simulink model "pmsm1"  (Simulink 7.0)
settings: Solver=ode23tb  StartTime=0.0  StopTime=1  MaxStep=1e-3  RelTol=1e-3
libraries: powerlib x12
settings Model: Creator=vegetable  LastModifiedBy=vegetable
settings OptimizationCC: InitFltsAndDblsToZero=off
settings DebuggingCC: SaveWithParameterizedLinksMsg=none  FcnCallInpInsideContextMsg=Enable All  StrictBusMsg=ErrorLevel1
settings HardwareCC: TargetHWDeviceType=32-bit Generic
settings GRTTargetCC: TargetFcnLib=ansi_tfl_tmw.mat

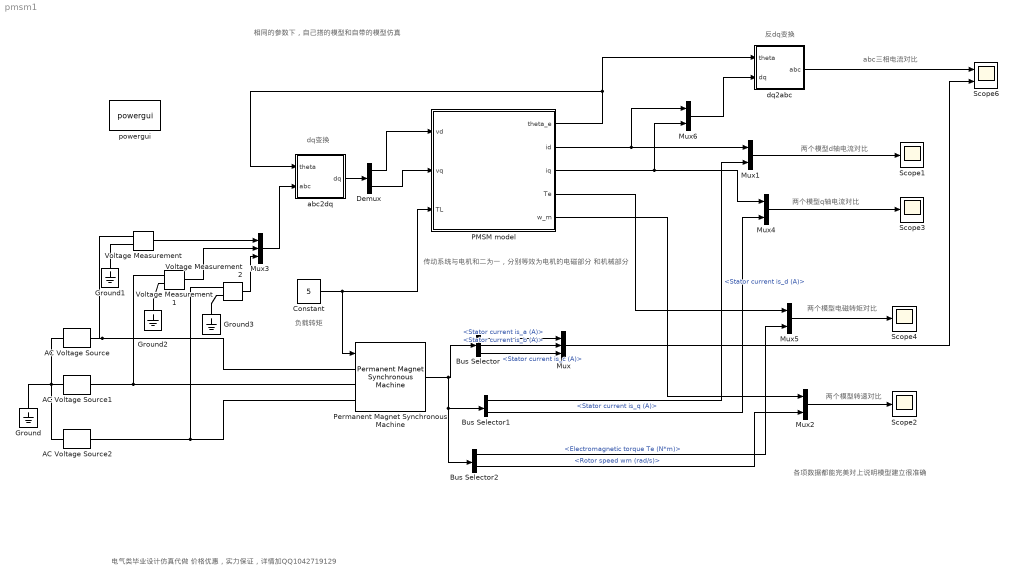
== system pmsm1 ==
  note: 电气类毕业设计仿真代做 价格优惠，实力保证，详情加QQ1042719129
  note: 反dq变换
  note: dq变换
  note: 相同的参数下，自己搭的模型和自带的模型仿真
  note: 传动系统与电机和二为一，分别等效为电机的电磁部分
      | 和机械部分
  note: 各项数据都能完美对上说明模型建立很准确
  note: abc三相电流对比
  note: 负载转矩
  note: 两个模型转速对比
  note: 两个模型电磁转矩对比
  note: 两个模型q轴电流对比
  note: 两个模型d轴电流对比
  AC Voltage Source : powerlib/Electrical Sources/AC Voltage Source  Amplitude=100  Phase=0  Frequency=60  SampleTime=0  Measurements=None
  AC Voltage Source1 : powerlib/Electrical Sources/AC Voltage Source  Amplitude=100  Phase=-120  Frequency=60  SampleTime=0  Measurements=None
  AC Voltage Source2 : powerlib/Electrical Sources/AC Voltage Source  Amplitude=100  Phase=120  Frequency=60  SampleTime=0  Measurements=None
  Bus Selector : BusSelector  OutputSignals=Stator current is_a (A),Stator current is_b (A),Stator current is_c (A)
  Bus Selector1 : BusSelector  OutputSignals=Stator current is_d (A),Stator current is_q (A)
  Bus Selector2 : BusSelector  OutputSignals=Electromagnetic torque Te (N*m),Rotor speed wm (rad/s)
  Constant : Constant  Value=5
  Demux : Demux  Outputs=2
  Ground{,1..3} (4 alike) : powerlib/Elements/Ground  Orientation=down  LConnTagsString=a
  Mux : Mux  Inputs=3
  Mux{1..2,4..6} (5 alike) : Mux  Inputs=2
  Mux3 : Mux  Inputs=3
  "PMSM model " : Subsystem  mask{Ld=0.0085, Lq=0.0085, Ra=2.875, J=8e-4, fai=0.175, p=60}
      mask prompts: Ld "d轴电感"; Lq "q轴电感"; Ra "电枢电阻"; J "转动惯量"; fai "磁链"; p "极对数"
  Permanent Magnet Synchronous Machine : powerlib/Machines/Permanent Magnet Synchronous Machine  NbPhases=3  FluxDistribution=Sinusoidal  RotorType=Round  MechanicalLoad=Torque Tm  PresetModel=No  ShowDetailedParameters=on  Resistance=2.875  Inductance=8.5e-3  dqInductances=[8.5e-3,8.5e-3]  La=0.0085  MachineConstant=Flux linkage established by magnets (V.s)  Flux=0.175  VoltageCst=1904.4893  TorqueCst=15.75  Flat=120  Mechanical=[8e-4 0.0003035 60 0]  PolePairs=60  InitialConditions=[0,0, 0,0]  InitialConditions5ph=[0 0 0 0 0 0]  TsPowergui=0  TsBlock=-1  RefAngle=90 degrees behind phase A axis (modified Park)
  Scope{1..4} (4 alike) : Scope
      Scope2 settings: SaveName=ScopeData2
      Scope3 settings: SaveName=ScopeData3
      Scope4 settings: SaveName=ScopeData4
  Scope6 : Scope  NumInputPorts=2
      settings: YMin=-5~-5  YMax=5~5  SaveName=ScopeData6
  Voltage Measurement : powerlib/Measurements/Voltage Measurement  PhasorSimulation=off  OutputType=Complex  PSBequivalent=0
  Voltage Measurement1 : powerlib/Measurements/Voltage Measurement  PhasorSimulation=off  OutputType=Complex  PSBequivalent=0
  Voltage Measurement2 : powerlib/Measurements/Voltage Measurement  PhasorSimulation=off  OutputType=Complex  PSBequivalent=0
  abc2dq : Subsystem
  dq2abc : Subsystem
  powergui : powerlib/powergui  Priority=1  SimulationMode=Continuous  SolverType=Tustin  SampleTime=50e-6  frequency=60  SPID=off  DisableSnubberDevices=off  DisableRonSwitches=off  DisableVfSwitches=off  SwTol=0  Interpol=off  DisplayEquations=off  FunctionMessages=off  frequencyindice=60  Pbase=100e6  ErrMax=1e-4  Iterations=50  UnitsV=kV  UnitsW=MW  echomessages=off  HookPort=off  EnableUseOfTLC=off  x0status=blocks  RestoreLinks=warning  ResistiveCurrentMeasurement=off  Ylog=off  Xlog=on  ShowGrid=off  save=off  variable=ZData  ZoomFFT=off  StartTime=0.0  cycles=1  DisplayStyle=1  FreqAxis=off  MaxFrequency=1000  frequencyindicesteady=1  display=off  methode=off
  wires:
  Permanent Magnet Synchronous Machine/1 -> Bus Selector2/1, Bus Selector1/1, Bus Selector/1
  Bus Selector/1 -> Mux/1  "<Stator current is_a (A)>"
  Mux/1 -> Scope6/2
  Mux1/1 -> Scope1/1
  Mux2/1 -> Scope2/1
  Constant/1 -> Permanent Magnet Synchronous Machine/1, "PMSM model "/3(TL)
  Voltage Measurement/1 -> Mux3/1
  Voltage Measurement1/1 -> Mux3/2
  Voltage Measurement2/1 -> Mux3/3
  Mux3/1 -> abc2dq/2(abc)
  abc2dq/1(dq) -> Demux/1
  Demux/1 -> "PMSM model "/1(vd)
  Demux/2 -> "PMSM model "/2(vq)
  "PMSM model "/1(theta_e) -> dq2abc/1(theta), abc2dq/1(theta)
  Bus Selector/2 -> Mux/2  "<Stator current is_b (A)>"
  Bus Selector/3 -> Mux/3  "<Stator current is_c (A)>"
  "PMSM model "/2(id) -> Mux6/1, Mux1/1
  Bus Selector1/1 -> Mux1/2  "<Stator current is_d (A)>"
  "PMSM model "/3(iq) -> Mux6/2, Mux4/1
  Bus Selector1/2 -> Mux4/2  "<Stator current is_q (A)>"
  Mux4/1 -> Scope3/1
  "PMSM model "/4(Te) -> Mux5/1
  Bus Selector2/1 -> Mux5/2  "<Electromagnetic torque Te (N*m)>"
  Mux5/1 -> Scope4/1
  "PMSM model "/5(w_m) -> Mux2/1
  Bus Selector2/2 -> Mux2/2  "<Rotor speed wm (rad/s)>"
  dq2abc/1(abc) -> Scope6/1
  Mux6/1 -> dq2abc/2(dq)
  connections:
  AC Voltage Source/LConn1 -- Ground/LConn1 -- AC Voltage Source1/LConn1 -- AC Voltage Source2/LConn1
  AC Voltage Source/RConn1 -- Permanent Magnet Synchronous Machine/LConn1 -- Voltage Measurement/LConn1
  AC Voltage Source1/RConn1 -- Voltage Measurement1/LConn1 -- Permanent Magnet Synchronous Machine/LConn2
  AC Voltage Source2/RConn1 -- Permanent Magnet Synchronous Machine/LConn3 -- Voltage Measurement2/LConn1
  Ground1/LConn1 -- Voltage Measurement/LConn2
  Ground2/LConn1 -- Voltage Measurement1/LConn2
  Ground3/LConn1 -- Voltage Measurement2/LConn2

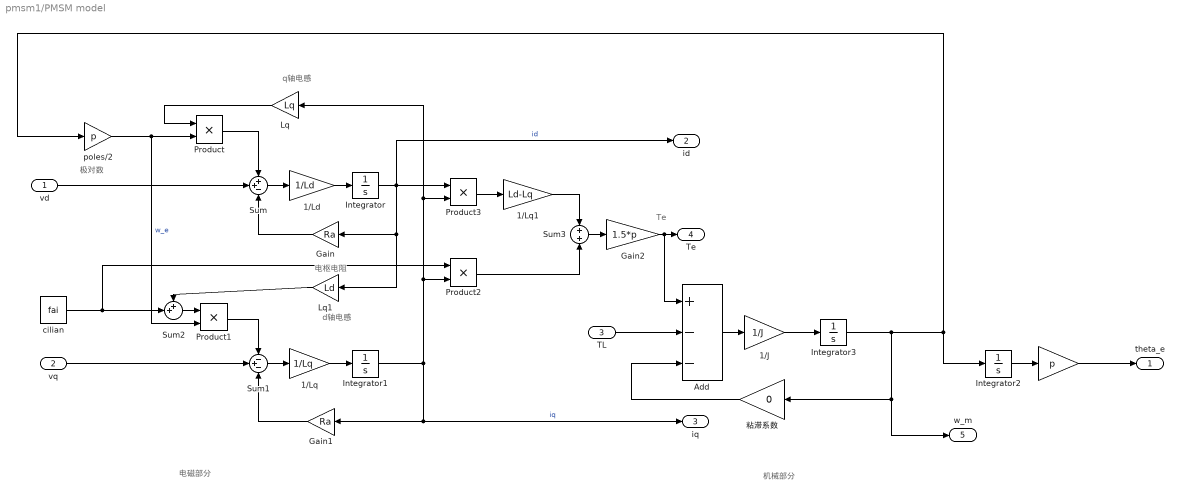
== system pmsm1/PMSM model  ==
  note: 机械部分
  note: 电磁部分
  note: q轴电感
  note: d轴电感
  note: 电枢电阻
  note: 极对数
  note: Te
  vd : Inport
  vq : Inport  Port=2
  TL : Inport  Port=3
  "  " : Gain  Gain=p
  1/J : Gain  Gain=1/J
  1/Ld : Gain  Gain=1/Ld  SaturateOnIntegerOverflow=on
  1/Lq : Gain  Gain=1/Lq  SaturateOnIntegerOverflow=on
  1/Lq1 : Gain  Gain=Ld-Lq  SaturateOnIntegerOverflow=on
  Add : Sum  Inputs=+--
  Gain : Gain  Orientation=left  Gain=Ra  SaturateOnIntegerOverflow=on
  Gain1 : Gain  Orientation=left  Gain=Ra  SaturateOnIntegerOverflow=on
  Gain2 : Gain  Gain=1.5*p  SaturateOnIntegerOverflow=on
  Integrator{,1..3} (4 alike) : Integrator
  Lq : Gain  Orientation=left  Gain=Lq  SaturateOnIntegerOverflow=on
  Lq1 : Gain  Orientation=left  Gain=Ld  SaturateOnIntegerOverflow=on
  Product{,1..3} (4 alike) : Product  SaturateOnIntegerOverflow=on  InputSameDT=on
  Sum : Sum  Inputs=++-  SaturateOnIntegerOverflow=on  InputSameDT=on
  Sum1 : Sum  Inputs=-+-  SaturateOnIntegerOverflow=on  InputSameDT=on
  Sum2 : Sum  Inputs=++|  SaturateOnIntegerOverflow=on  InputSameDT=on
  Sum3 : Sum  SaturateOnIntegerOverflow=on  InputSameDT=on
  cilian : Constant  Value=fai
  poles/2 : Gain  Gain=p  SaturateOnIntegerOverflow=on
  粘滞系数 : Gain  Orientation=left  Gain=0  SaturateOnIntegerOverflow=on
  theta_e : Outport
  id : Outport  Port=2
  iq : Outport  Port=3
  Te : Outport  Port=4
  w_m : Outport  Port=5
  wires:
  Gain/1 -> Sum/3
  vq/1 -> Sum1/2
  Gain1/1 -> Sum1/3
  Integrator/1 -> Gain/1, Lq1/1, Product3/1, id/1  "id"
  Product1/1 -> Sum1/1
  Product/1 -> Sum/1
  Lq/1 -> Product/1
  vd/1 -> Sum/2
  Sum1/1 -> 1/Lq/1
  Sum/1 -> 1/Ld/1
  Sum3/1 -> Gain2/1
  poles/2/1 -> Product/2, Product1/2  "w_e"
  1/Ld/1 -> Integrator/1
  1/Lq/1 -> Integrator1/1
  Integrator1/1 -> Product2/2, Product3/2, Lq/1, Gain1/1, iq/1  "iq"
  Sum2/1 -> Product1/1
  cilian/1 -> Sum2/2, Product2/1
  Product3/1 -> 1/Lq1/1
  Product2/1 -> Sum3/2
  1/Lq1/1 -> Sum3/1
  Lq1/1 -> Sum2/1
  "  "/1 -> theta_e/1
  1/J/1 -> Integrator3/1
  Integrator3/1 -> 粘滞系数/1, w_m/1, poles/2/1, Integrator2/1
  Add/1 -> 1/J/1
  Integrator2/1 -> "  "/1
  Gain2/1 -> Add/1, Te/1
  TL/1 -> Add/2
  粘滞系数/1 -> Add/3

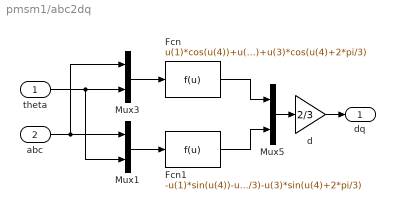
== system pmsm1/abc2dq ==
  theta : Inport
  abc : Inport  Port=2
  Fcn : Fcn  Expr=u(1)*cos(u(4))+u(2)*cos(u(4)-2*pi/3)+u(3)*cos(u(4)+2*pi/3)
  Fcn1 : Fcn  Expr=-u(1)*sin(u(4))-u(2)*sin(u(4)-2*pi/3)-u(3)*sin(u(4)+2*pi/3)
  Mux1 : Mux  Inputs=2
  Mux3 : Mux  Inputs=2
  Mux5 : Mux  Inputs=2
  d : Gain  Gain=2/3
  dq : Outport
  wires:
  Mux3/1 -> Fcn/1
  Fcn/1 -> Mux5/1
  Mux5/1 -> d/1
  Mux1/1 -> Fcn1/1
  Fcn1/1 -> Mux5/2
  abc/1 -> Mux1/1, Mux3/1
  theta/1 -> Mux3/2, Mux1/2
  d/1 -> dq/1

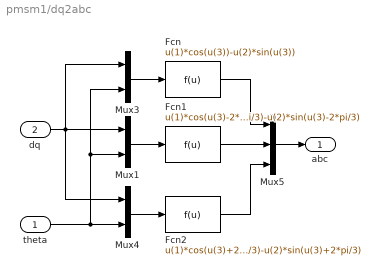
== system pmsm1/dq2abc ==
  theta : Inport
  dq : Inport  Port=2
  Fcn : Fcn  Expr=u(1)*cos(u(3))-u(2)*sin(u(3))
  Fcn1 : Fcn  Expr=u(1)*cos(u(3)-2*pi/3)-u(2)*sin(u(3)-2*pi/3)
  Fcn2 : Fcn  Expr=u(1)*cos(u(3)+2*pi/3)-u(2)*sin(u(3)+2*pi/3)
  Mux1 : Mux  Inputs=2
  Mux3 : Mux  Inputs=2
  Mux4 : Mux  Inputs=2
  Mux5 : Mux  Inputs=3
  abc : Outport
  wires:
  theta/1 -> Mux1/2, Mux3/2, Mux4/2
  Fcn2/1 -> Mux5/3
  Fcn1/1 -> Mux5/2
  Mux1/1 -> Fcn1/1
  Mux5/1 -> abc/1
  Fcn/1 -> Mux5/1
  Mux4/1 -> Fcn2/1
  Mux3/1 -> Fcn/1
  dq/1 -> Mux3/1, Mux1/1, Mux4/1
